simulink model "SMC"  (R2020b)
settings: Solver=ode45  StartTime=0.0  StopTime=10.0  MaxStep=0.02  RelTol=1e-3  EnableMultiTasking=on
undefined symbols (not defined in the file): a, b, cond_init, delta, g, Kc, l, m
libraries: simulink x1
settings Model: Creator=Administrador  LastModifiedBy=andre
settings DataIOCC: LimitDataPoints=on  SaveFormat=Array  SignalLoggingSaveFormat=ModelDataLogs  ReturnWorkspaceOutputs=off
settings OptimizationCC: ExpressionDepthLimit=2147483647  InitFltsAndDblsToZero=on  LifeSpan=inf
settings DebuggingCC: UnderspecifiedInitializationDetection=Classic  MergeDetectMultiDrivingBlocksExec=none  SolverPrmCheckMsg=warning  FcnCallInpInsideContextMsg=warning  StateNameClashWarn=warning  SFUnexpectedBacktrackingDiag=warning  SFNoUnconditionalDefaultTransitionDiag=warning  SFExecutionAtInitializationDiag=none  ArithmeticOperatorsInVariantConditions=warning
settings HardwareCC: ProdBitPerPointer=32  ProdBitPerSizeT=32  ProdBitPerPtrDiffT=32  ProdLargestAtomicFloat=None  ProdIntDivRoundTo=Undefined  ProdEndianess=Unspecified  ProdWordSize=32  ProdHWDeviceType=32-bit Generic
settings ModelReferenceCC: PropagateSignalLabelsOutOfModel=off
settings SFSimCC: SimUseLocalCustomCode=off  CustomCodeUndefinedFunction=UseInterfaceOnly
settings RTWCC: RTWUseLocalCustomCode=off
settings CodeAppCC: StateflowObjectComments=on
settings GRTTargetCC: TargetLangStandard=C89/C90 (ANSI)  CombineOutputUpdateFcns=off  GRTInterface=on
settings ConfigComp: CovMetricSettings=dw  CovSaveCumulativeToWorkspaceVar=on  CovSaveSingleToWorkspaceVar=on  CovExternalEMLEnable=off

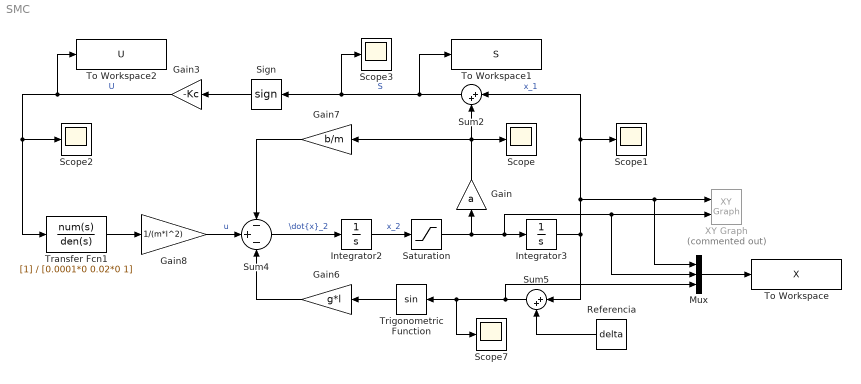
== system SMC ==
  Gain : Gain  Gain=a
  Gain3 : Gain  Gain=-Kc
  Gain6 : Gain  Gain=g*l
  Gain7 : Gain  Gain=b/m
  Gain8 : Gain  Gain=1/(m*l^2)
  Integrator2 : Integrator
  Integrator3 : Integrator  InitialCondition=cond_init
  Mux : Mux  Inputs=3
  Referencia : Constant  Value=delta
  Saturation : Saturate  UpperLimit=2*pi  LowerLimit=-2*pi
  Scope{,1..3,7} (5 alike) : Scope
  Sign : Signum  ZeroCross=off
  Sum2 : Sum  Inputs=|++
  Sum4 : Sum  Inputs=-+-
  Sum5 : Sum  Inputs=|++
  To Workspace : ToWorkspace  VariableName=X  SaveFormat=Timeseries  SampleTime=-1
  To Workspace1 : ToWorkspace  VariableName=S  SaveFormat=Timeseries  SampleTime=-1
  To Workspace2 : ToWorkspace  VariableName=U  SaveFormat=Timeseries  SampleTime=-1
  Transfer Fcn1 : TransferFcn  Denominator=[0.0001*0 0.02*0 1]
  Trigonometric Function : Trigonometry
  XY Graph : simulink/Sinks/XY Graph  Commented=on  xmin=-3  xmax=1  ymin=-1  ymax=5  st=-1
  wires:
  Sum2/1 -> To Workspace1/1, Scope3/1, Sign/1  "S"
  Sign/1 -> Gain3/1
  Gain3/1 -> To Workspace2/1, Transfer Fcn1/1, Scope2/1  "U"
  Integrator3/1 -> Mux/1, XY Graph/1, Sum2/1, Scope1/1, Sum5/1  "x_1"
  Referencia/1 -> Sum5/2
  Gain7/1 -> Sum4/1
  Trigonometric Function/1 -> Gain6/1
  Sum4/1 -> Integrator2/1  "\\dot{x}_2"
  Gain8/1 -> Sum4/2  "u"
  Sum5/1 -> Mux/3, Trigonometric Function/1, Scope7/1
  Integrator2/1 -> Saturation/1  "x_2"
  Gain6/1 -> Sum4/3
  Gain/1 -> Gain7/1, Scope/1, Sum2/2
  Mux/1 -> To Workspace/1
  Transfer Fcn1/1 -> Gain8/1
  Saturation/1 -> Mux/2, XY Graph/2, Integrator3/1, Gain/1
